simulink model "simulation"  (R2014a)
settings: Solver=ode45  StartTime=0.0  StopTime=10  RelTol=1e-3
settings Model: Creator=usmankhan  LastModifiedBy=usmankhan

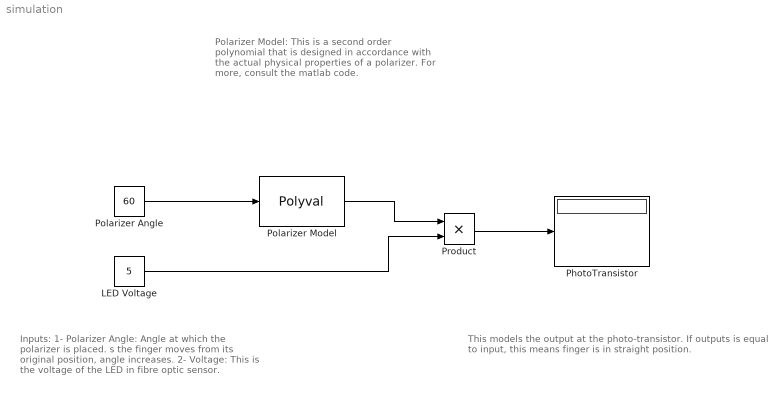
== system simulation ==
  note: Polarizer Model:
      |
      | This is a second order polynomial
      | that is designed in accordance with
      | the actual physical properties of a
      | polarizer. For more, consult the
      | matlab code.
  note: Inputs:
      |
      | 1- Polarizer Angle: Angle at which
      | the polarizer is placed. s the finger
      | moves from its original position, angle
      | increases.
      |
      | 2- Voltage: This is the voltage of the
      | LED in fibre optic sensor.
  note: This models the output at the photo-transistor.
      | If outputs is equal to input, this means finger
      | is in straight position.
  " LED Voltage" : Constant  Value=5  SampleTime=Inf
  PhotoTransistor : Display
  Polarizer Angle : Constant  Value=60  SampleTime=Inf
  Polarizer Model : Polyval  Coefs=[-0.0001,-0.0024, 1.0208]
  Product : Product
  wires:
  Polarizer Angle/1 -> Polarizer Model/1
  Polarizer Model/1 -> Product/1
  " LED Voltage"/1 -> Product/2
  Product/1 -> PhotoTransistor/1
